simulink model "ex2"  (Simulink 6.0)
settings: Solver=ode45  StartTime=0.0  StopTime=10.0  RelTol=1e-3
undefined symbols (not defined in the file or in its folder): functieg
settings Model: LastModifiedBy=student

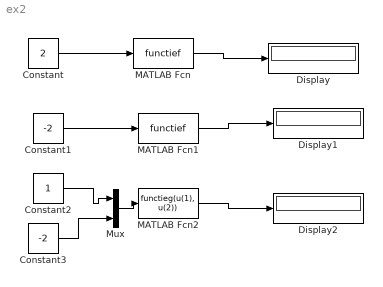
== system ex2 ==
  Constant : Constant  Value=2
  Constant1 : Constant  Value=-2
  Constant2 : Constant
  Constant3 : Constant  Value=-2
  Display : Display
  Display1 : Display
  Display2 : Display
  MATLAB Fcn : MATLABFcn  MATLABFcn=functief
  MATLAB Fcn1 : MATLABFcn  MATLABFcn=functief
  MATLAB Fcn2 : MATLABFcn  MATLABFcn=functieg(u(1), u(2))
  Mux : Mux  Inputs=2
  wires:
  Constant/1 -> MATLAB Fcn/1
  MATLAB Fcn/1 -> Display/1
  Constant1/1 -> MATLAB Fcn1/1
  MATLAB Fcn1/1 -> Display1/1
  Constant2/1 -> Mux/1
  MATLAB Fcn2/1 -> Display2/1
  Constant3/1 -> Mux/2
  Mux/1 -> MATLAB Fcn2/1
